simulink model "manipulator"  (R2019a)
settings: Solver=FixedStepAuto  StartTime=0.0  StopTime=30  FixedStep=0.01  RelTol=1e-3
values from neighbouring files (symbols this model uses):
  dTheta0 = 0    [setCoef.m]
  Theta0 = 45*pi/180    (= 0.785398163397)    [setCoef.m]
settings Model: Creator=Петр  LastModifiedBy=petr
settings DataIOCC: ReturnWorkspaceOutputs=off
settings DebuggingCC: PregeneratedLibrarySubsystemCodeDiagnostic=none  ArithmeticOperatorsInVariantConditions=warning
settings SFSimCC: SimUseLocalCustomCode=off
settings RTWCC: RTWUseLocalCustomCode=off

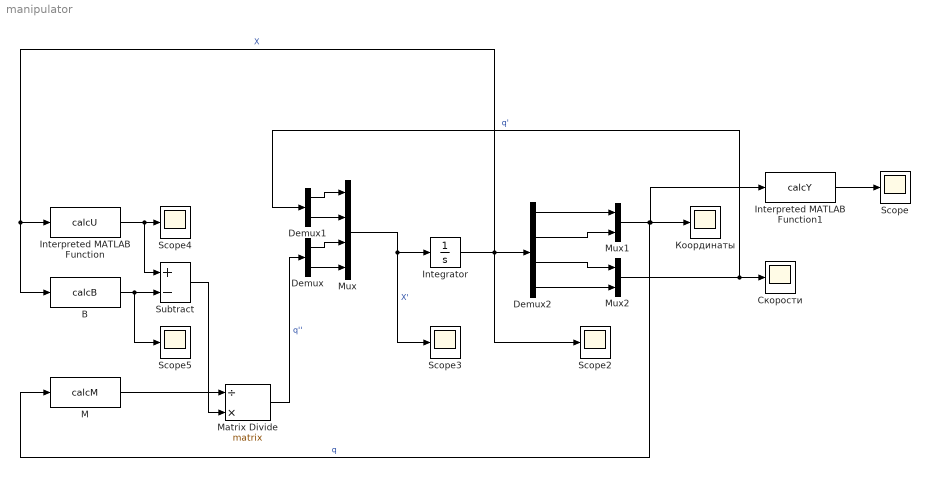
== system manipulator ==
  B : MATLABFcn  MATLABFcn=calcB  OutputDimensions=[2 1]  Output1D=off
  Demux : Demux  Outputs=2
  Demux1 : Demux  Outputs=2
  Demux2 : Demux
  Integrator : Integrator  InitialCondition=[0; Theta0; 0; dTheta0]  UpperSaturationLimit=10000  LowerSaturationLimit=-10000
  Interpreted MATLAB Function : MATLABFcn  MATLABFcn=calcU
  Interpreted MATLAB Function1 : MATLABFcn  MATLABFcn=calcY
  M : MATLABFcn  MATLABFcn=calcM  OutputDimensions=[2 2]  Output1D=off
  Matrix Divide : Product  Inputs=/*  Multiplication=Matrix(*)
  Mux : Mux
  Mux1 : Mux  Inputs=2
  Mux2 : Mux  Inputs=2
  Scope{,2..5} (5 alike) : Scope
  Subtract : Sum  Inputs=+-
  Координаты : Scope
  Скорости : Scope
  wires:
  M/1 -> Matrix Divide/1
  Matrix Divide/1 -> Demux/1  "q''"
  Demux1/1 -> Mux/1
  Demux1/2 -> Mux/2
  Demux/1 -> Mux/3
  Demux/2 -> Mux/4
  Mux/1 -> Scope3/1, Integrator/1  "X'"
  Integrator/1 -> Interpreted MATLAB Function/1, B/1, Scope2/1, Demux2/1  "X"
  Demux2/1 -> Mux1/1
  Demux2/2 -> Mux1/2
  Demux2/4 -> Mux2/2
  Demux2/3 -> Mux2/1
  Mux1/1 -> Interpreted MATLAB Function1/1, Координаты/1, M/1  "q"
  Mux2/1 -> Demux1/1, Скорости/1  "q'"
  Subtract/1 -> Matrix Divide/2
  B/1 -> Scope5/1, Subtract/2
  Interpreted MATLAB Function/1 -> Scope4/1, Subtract/1
  Interpreted MATLAB Function1/1 -> Scope/1
